simulink model "PR9"  (R2019b)
settings: Solver=VariableStepAuto  StartTime=0.0  StopTime=200  RelTol=1e-3  EnableMultiTasking=on
libraries: simulink x1
settings Model: Creator=Zachary  LastModifiedBy=bhisma
settings DataIOCC: LimitDataPoints=on  ReturnWorkspaceOutputs=off
settings OptimizationCC: LifeSpan=inf
settings DebuggingCC: AllowSymbolicDim=off  SFUnexpectedBacktrackingDiag=warning  SFNoUnconditionalDefaultTransitionDiag=warning  SFExecutionAtInitializationDiag=none  ArithmeticOperatorsInVariantConditions=warning
settings ModelReferenceCC: PropagateSignalLabelsOutOfModel=off
settings SFSimCC: SimUseLocalCustomCode=off  CustomCodeUndefinedFunction=UseInterfaceOnly
settings RTWCC: RTWUseLocalCustomCode=off
settings CodeAppCC: StateflowObjectComments=on
settings GRTTargetCC: TargetLangStandard=C89/C90 (ANSI)
settings ConfigComp: CovMetricSettings=dw  CovHtmlReporting=on  CovSaveCumulativeToWorkspaceVar=on  CovSaveSingleToWorkspaceVar=on  CovExternalEMLEnable=off

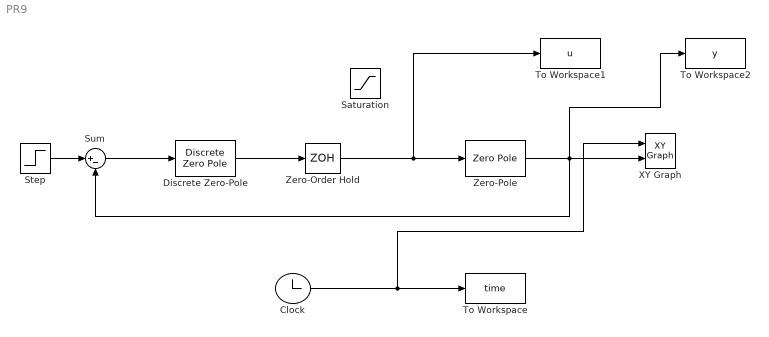
== system PR9 ==
  Clock : Clock
  Discrete Zero-Pole : DiscreteZeroPole  Zeros=[]  Poles=[]  Gain=8.1  SampleTime=0.1
  Saturation : Saturate  UpperLimit=10  LowerLimit=-10
  Step : Step  SampleTime=0.1
  Sum : Sum  Inputs=|+-
  To Workspace : ToWorkspace  VariableName=time  SaveFormat=Timeseries  SampleTime=-1
  To Workspace1 : ToWorkspace  VariableName=u  SaveFormat=Timeseries  SampleTime=-1
  To Workspace2 : ToWorkspace  VariableName=y  SaveFormat=Timeseries  SampleTime=-1
  XY Graph : simulink/Sinks/XY Graph  xmin=0  xmax=200  ymin=-5  ymax=5  st=-1
  Zero-Order Hold : ZeroOrderHold  SampleTime=0.1
  Zero-Pole : ZeroPole  Zeros=[]  Poles=[0 -0.4]
  wires:
  Discrete Zero-Pole/1 -> Zero-Order Hold/1
  Zero-Pole/1 -> Sum/2, To Workspace2/1, XY Graph/2
  Clock/1 -> To Workspace/1, XY Graph/1
  Sum/1 -> Discrete Zero-Pole/1
  Step/1 -> Sum/1
  Zero-Order Hold/1 -> To Workspace1/1, Zero-Pole/1
